simulink model "mw_spectrumanalyser"  (R2020a)
settings: Solver=VariableStepAuto  StartTime=0.0  StopTime=100000/256e6  RelTol=1e-3
InitFcn:
  | fs = 256e6;
undefined symbols (not defined in the file or in its folder): designMultirateFIR
libraries: hdlsllib x109, simulink x50, dsphdlxfrm x8, dspmlti4 x6, dspswit3 x4, dspsigops x2, dspsigattribs x2
(part 1 of 3)
settings Model: Creator=david  LastModifiedBy=david
settings OptimizationCC: BlockReduction=off  ConditionallyExecuteInputs=off  DefaultParameterBehavior=Inlined
settings DebuggingCC: AlgebraicLoopMsg=error
settings HardwareCC: ProdBitPerPointer=32  ProdBitPerSizeT=32  ProdBitPerPtrDiffT=32  ProdLargestAtomicFloat=None  ProdIntDivRoundTo=Undefined  ProdEndianess=Unspecified  ProdWordSize=32  ProdHWDeviceType=ASIC/FPGA->ASIC/FPGA  TargetBitPerPointer=64  TargetBitPerSizeT=64  TargetBitPerPtrDiffT=64  TargetLongLongMode=on  TargetIntDivRoundTo=Zero  TargetEndianess=LittleEndian  TargetWordSize=64  TargetHWDeviceType=Custom Processor->MATLAB Host Computer  ProdEqTarget=off

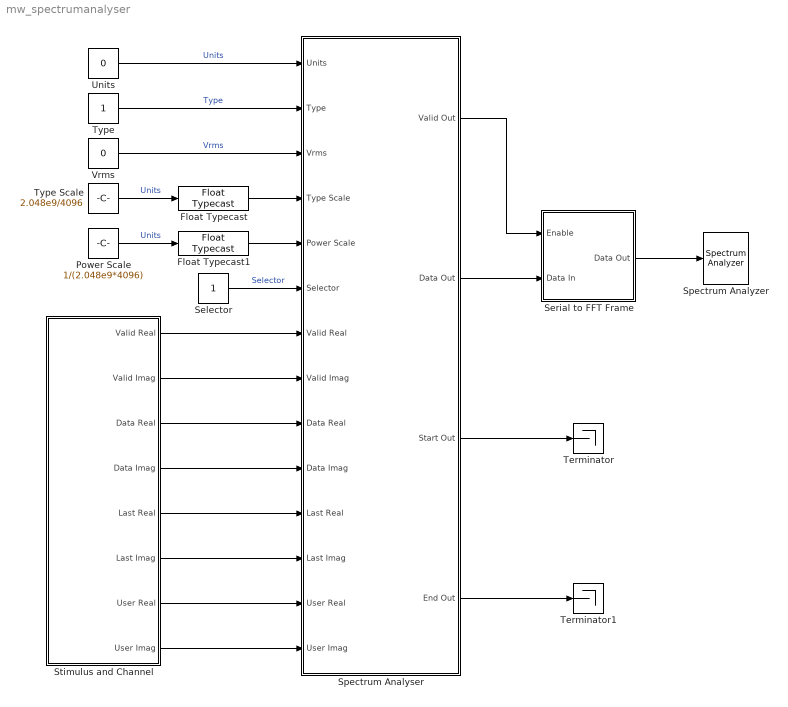
== system mw_spectrumanalyser ==
  Float Typecast : FloatTypecast
  Float Typecast1 : FloatTypecast
  Power Scale : Constant  Value=1/(2.048e9*4096)  OutDataTypeStr=single  SampleTime=-1
  Selector : Constant  OutDataTypeStr=uint32  SampleTime=-1
  Serial to FFT Frame : Subsystem  mask{N=4096}
      mask prompts: N "FFT Size:"
      mask DialogControl DescGroupVar Prompt: Serial to FFT Frame
      mask DialogControl DescTextVar Prompt: This block converts serial FFT data to a frame of FFT data. An FFT shift is applied to correct for out of order FFT data.
      mask DialogControl ParameterGroupVar Prompt: Main
  Spectrum Analyzer : SpectrumAnalyzer  IsFrequencyInputMode=1
  Spectrum Analyser : Subsystem  TreatAsAtomicUnit=on
  Stimulus and Channel : Subsystem
  Terminator : Terminator
  Terminator1 : Terminator
  Type : Constant  OutDataTypeStr=uint32  SampleTime=-1
  Type Scale : Constant  Value=2.048e9/4096  OutDataTypeStr=single  SampleTime=-1
  Units : Constant  Value=0  OutDataTypeStr=uint32  SampleTime=-1
  Vrms : Constant  Value=0  OutDataTypeStr=uint32  SampleTime=-1
  wires:
  Spectrum Analyser/3(Start Out) -> Terminator/1
  Spectrum Analyser/4(End Out) -> Terminator1/1
  Spectrum Analyser/2(Data Out) -> Serial to FFT Frame/2(Data In)
  Spectrum Analyser/1(Valid Out) -> Serial to FFT Frame/1(Enable)
  Serial to FFT Frame/1(Data Out) -> Spectrum Analyzer/1
  Stimulus and Channel/1(Valid Real) -> Spectrum Analyser/7(Valid Real)
  Stimulus and Channel/2(Valid Imag) -> Spectrum Analyser/8(Valid Imag)
  Stimulus and Channel/3(Data Real) -> Spectrum Analyser/9(Data Real)
  Stimulus and Channel/4(Data Imag) -> Spectrum Analyser/10(Data Imag)
  Vrms/1 -> Spectrum Analyser/3(Vrms)  "Vrms"
  Type/1 -> Spectrum Analyser/2(Type)  "Type"
  Units/1 -> Spectrum Analyser/1(Units)  "Units"
  Type Scale/1 -> Float Typecast/1  "Units"
  Float Typecast/1 -> Spectrum Analyser/4(Type Scale)
  Float Typecast1/1 -> Spectrum Analyser/5(Power Scale)
  Power Scale/1 -> Float Typecast1/1  "Units"
  Stimulus and Channel/5(Last Real) -> Spectrum Analyser/11(Last Real)
  Stimulus and Channel/6(Last Imag) -> Spectrum Analyser/12(Last Imag)
  Stimulus and Channel/7(User Real) -> Spectrum Analyser/13(User Real)
  Stimulus and Channel/8(User Imag) -> Spectrum Analyser/14(User Imag)
  Selector/1 -> Spectrum Analyser/6(Selector)  "Selector"

== system mw_spectrumanalyser/Serial to FFT Frame ==
  Enable : Inport
  Data In : Inport  Port=2
  Enabled Subsystem2 : Subsystem  TreatAsAtomicUnit=on
  Float Typecast : FloatTypecast
  Matrix Concatenate2 : Concatenate  Mode=Multidimensional array
  Selector1 : Selector  InputPortWidth=N  IndexOptions=Index vector (dialog)  Indices=[1:1:N/2+1]  OutputSizes=1
  Selector4 : Selector  InputPortWidth=N  IndexOptions=Index vector (dialog)  Indices=[N/2+2:1:N]  OutputSizes=1
  Data Out : Outport
  wires:
  Float Typecast/1 -> Data Out/1
  Selector4/1 -> Matrix Concatenate2/1
  Selector1/1 -> Matrix Concatenate2/2
  Matrix Concatenate2/1 -> Float Typecast/1
  Data In/1 -> Enabled Subsystem2/1(Data In)
  Enable/1 -> Enabled Subsystem2/Enable
  Enabled Subsystem2/1(Data Out) -> Selector1/1, Selector4/1

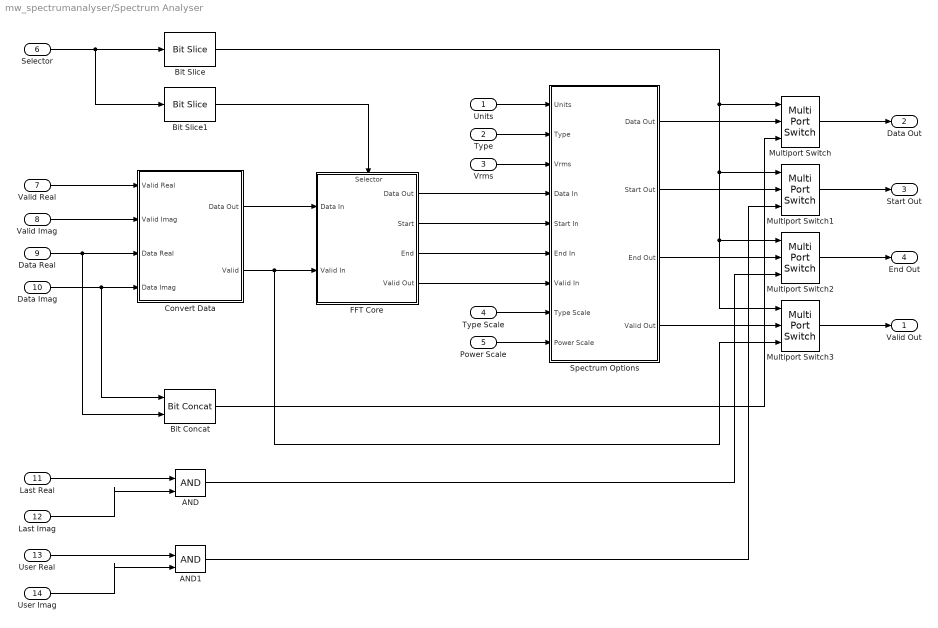
== system mw_spectrumanalyser/Spectrum Analyser ==
  Units : Inport
  Type : Inport  Port=2
  Vrms : Inport  Port=3
  Type Scale : Inport  Port=4
  Power Scale : Inport  Port=5
  Selector : Inport  Port=6
  Valid Real : Inport  Port=7
  Valid Imag : Inport  Port=8
  Data Real : Inport  Port=9
  Data Imag : Inport  Port=10
  Last Real : Inport  Port=11
  Last Imag : Inport  Port=12
  User Real : Inport  Port=13
  User Imag : Inport  Port=14
  AND : Logic  IconShape=distinctive  AllPortsSameDT=off  OutDataTypeStr=boolean
  AND1 : Logic  IconShape=distinctive  AllPortsSameDT=off  OutDataTypeStr=boolean
  Bit Concat : hdlsllib/Logic and Bit Operations/Bit Concat  numInputs=2
  Bit Slice : hdlsllib/Logic and Bit Operations/Bit Slice  lidx=8  ridx=8
      settings: SourceProductBaseCode=SL
  Bit Slice1 : hdlsllib/Logic and Bit Operations/Bit Slice  lidx=7  ridx=0
      settings: SourceProductBaseCode=SL
  Convert Data : Subsystem
  FFT Core : Subsystem  VariantControl=FFT
      settings: PortSchema="{\"entries\":[{\"content\":{\"sides\":[{\"content\":{\"connectorIds\":[\"In1\",\"In2\"]},\"type\":\"ConnectorPlacement.EquallySpacedRectSide\",\"uuid\":\"5a82c6db-67e2-4b0c-874b-00e78ac3fdee\"},{\"content\":{\"connectorIds\":[\"Out1\",\"Out2\",\"Out3\",\"Out4\"],\"side\":\"RIGHT\"},\"type\":\"ConnectorPlacement.EquallySpacedRectSide\",\"uuid\":\"dd11d034-f57b-4257-86c3-a224676007d8\"},{\"content\":{\"connectorIds\":[\"In3\"],\"side\":\"TOP\"},\"type\":\"ConnectorPlacement.EquallySpacedRectSide\",\"uuid\":\"15a5b623-5fad-4b26-a0b8-0856d140e740\"}]},\"type\":\"ConnectorPlacement.EquallySpacedConnector\",\"uuid\":\"f1901d0a-924b-44ce-aa2b-38fba4da21f9\"}],\"packageUris\":[\"http://schema.mathworks.com/mf0/Connector/19700101\"],\"version\":\"1.0\"}"
  Multiport Switch{,1..3} (4 alike) : MultiPortSwitch  DataPortOrder=Zero-based contiguous  Inputs=2  zeroidx=on
  Spectrum Options : Subsystem  VariantControl=Options
  Valid Out : Outport
  Data Out : Outport  Port=2
  Start Out : Outport  Port=3
  End Out : Outport  Port=4
  wires:
  FFT Core/4(Valid Out) -> Spectrum Options/7(Valid In)
  FFT Core/3(End) -> Spectrum Options/6(End In)
  FFT Core/2(Start) -> Spectrum Options/5(Start In)
  FFT Core/1(Data Out) -> Spectrum Options/4(Data In)
  Vrms/1 -> Spectrum Options/3(Vrms)
  Type/1 -> Spectrum Options/2(Type)
  Units/1 -> Spectrum Options/1(Units)
  Convert Data/1(Data Out) -> FFT Core/1(Data In)
  Data Imag/1 -> Bit Concat/1, Convert Data/4(Data Imag)
  Data Real/1 -> Bit Concat/2, Convert Data/3(Data Real)
  Valid Imag/1 -> Convert Data/2(Valid Imag)
  Valid Real/1 -> Convert Data/1(Valid Real)
  Type Scale/1 -> Spectrum Options/8(Type Scale)
  Power Scale/1 -> Spectrum Options/9(Power Scale)
  Spectrum Options/1(Data Out) -> Multiport Switch/2
  Multiport Switch/1 -> Data Out/1
  Spectrum Options/2(Start Out) -> Multiport Switch1/2
  Multiport Switch1/1 -> Start Out/1
  Spectrum Options/3(End Out) -> Multiport Switch2/2
  Multiport Switch2/1 -> End Out/1
  Spectrum Options/4(Valid Out) -> Multiport Switch3/2
  Multiport Switch3/1 -> Valid Out/1
  Selector/1 -> Bit Slice1/1, Bit Slice/1
  Last Real/1 -> AND/1
  Last Imag/1 -> AND/2
  User Real/1 -> AND1/1
  User Imag/1 -> AND1/2
  Bit Slice/1 -> Multiport Switch3/1, Multiport Switch2/1, Multiport Switch1/1, Multiport Switch/1
  Bit Concat/1 -> Multiport Switch/3
  Convert Data/2(Valid) -> Multiport Switch3/3, FFT Core/2(Valid In)
  AND/1 -> Multiport Switch2/3
  AND1/1 -> Multiport Switch1/3
  Bit Slice1/1 -> FFT Core/3(Selector)

== system mw_spectrumanalyser/Stimulus and Channel ==
  Channel : Subsystem
  Enable : Constant  OutDataTypeStr=boolean  SampleTime=-1
  Packet Size : Constant  Value=512  OutDataTypeStr=uint32  SampleTime=-1
  SSR Mode : Constant  Value=3  OutDataTypeStr=uint32  SampleTime=-1
  SSR Subset Converter Im : Subsystem  TreatAsAtomicUnit=on
  SSR Subset Converter Re : Subsystem  TreatAsAtomicUnit=on
  Transmitter : Subsystem  TreatAsAtomicUnit=on
  Value : Constant  Value=hex2dec('7FFF7FFF')  OutDataTypeStr=uint32  SampleTime=-1
  Valid Real : Outport
  Valid Imag : Outport  Port=2
  Data Real : Outport  Port=3
  Data Imag : Outport  Port=4
  Last Real : Outport  Port=5
  Last Imag : Outport  Port=6
  User Real : Outport  Port=7
  User Imag : Outport  Port=8
  wires:
  Enable/1 -> Transmitter/1(Enable)  "Enable"
  Transmitter/1(Valid) -> Channel/1(Valid)
  Transmitter/2(Data) -> Channel/2(Data)
  Value/1 -> Transmitter/2(Value)  "Value"
  Channel/2(Data Real) -> SSR Subset Converter Re/4(Data In)
  Channel/1(Valid Real) -> SSR Subset Converter Re/3(Valid In)
  SSR Mode/1 -> SSR Subset Converter Im/2(SSR Mode), SSR Subset Converter Re/2(SSR Mode)
  Packet Size/1 -> SSR Subset Converter Im/1(Packet Size), SSR Subset Converter Re/1(Packet Size)
  SSR Subset Converter Re/1(Valid Out) -> Valid Real/1
  SSR Subset Converter Re/2(Data Out) -> Data Real/1
  SSR Subset Converter Im/2(Data Out) -> Data Imag/1
  SSR Subset Converter Im/1(Valid Out) -> Valid Imag/1
  Channel/3(Valid Imag) -> SSR Subset Converter Im/3(Valid In)
  Channel/4(Data Imag) -> SSR Subset Converter Im/4(Data In)
  SSR Subset Converter Re/4(Last Out) -> Last Real/1
  SSR Subset Converter Im/4(Last Out) -> Last Imag/1
  SSR Subset Converter Re/3(User Out) -> User Real/1
  SSR Subset Converter Im/3(User Out) -> User Imag/1

== system mw_spectrumanalyser/Serial to FFT Frame/Enabled Subsystem2 ==
  Data In : Inport
  Enable : EnablePort
  Buffer : Buffer  N=N  OutputFrames=off
  Data Out : Outport
  wires:
  Buffer/1 -> Data Out/1
  Data In/1 -> Buffer/1

== system mw_spectrumanalyser/Spectrum Analyser/Convert Data ==
  Valid Real : Inport
  Valid Imag : Inport  Port=2
  Data Real : Inport  Port=3
  Data Imag : Inport  Port=4
  AND : Logic  IconShape=distinctive  AllPortsSameDT=off  OutDataTypeStr=boolean
  Data Type Conversion : DataTypeConversion  OutDataTypeStr=fixdt(1,16,15)  ConvertRealWorld=Stored Integer (SI)
  Data Type Conversion1 : DataTypeConversion  OutDataTypeStr=fixdt(1,16,15)  ConvertRealWorld=Stored Integer (SI)
  Real-Imag to Complex : RealImagToComplex
  Data Out : Outport
  Valid : Outport  Port=2
  wires:
  Real-Imag to Complex/1 -> Data Out/1
  AND/1 -> Valid/1
  Valid Real/1 -> AND/1
  Data Imag/1 -> Data Type Conversion1/1
  Data Type Conversion/1 -> Real-Imag to Complex/1
  Data Real/1 -> Data Type Conversion/1
  Data Type Conversion1/1 -> Real-Imag to Complex/2
  Valid Imag/1 -> AND/2

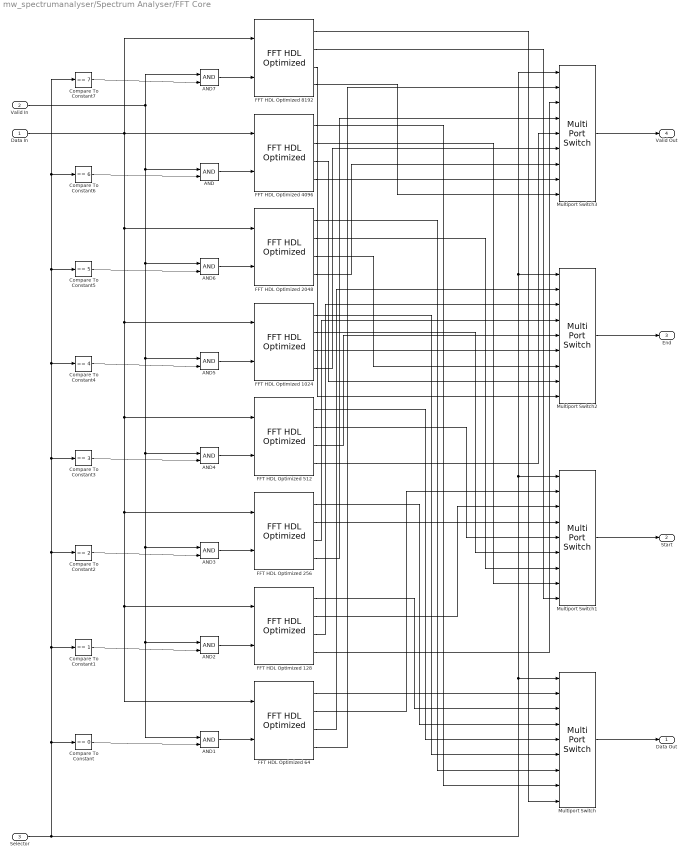
== system mw_spectrumanalyser/Spectrum Analyser/FFT Core ==
  Data In : Inport
  Valid In : Inport  Port=2
  Selector : Inport  Port=3
  AND{,1..7} (8 alike) : Logic  IconShape=distinctive  AllPortsSameDT=off  OutDataTypeStr=boolean
  Compare To Constant : simulink/Logic and Bit Operations/Compare To Constant  relop===  const=0  OutDataTypeStr=boolean
  Compare To Constant1 : simulink/Logic and Bit Operations/Compare To Constant  relop===  const=1  OutDataTypeStr=boolean
  Compare To Constant2 : simulink/Logic and Bit Operations/Compare To Constant  relop===  const=2  OutDataTypeStr=boolean
  Compare To Constant3 : simulink/Logic and Bit Operations/Compare To Constant  relop===  const=3  OutDataTypeStr=boolean
  Compare To Constant4 : simulink/Logic and Bit Operations/Compare To Constant  relop===  const=4  OutDataTypeStr=boolean
  Compare To Constant5 : simulink/Logic and Bit Operations/Compare To Constant  relop===  const=5  OutDataTypeStr=boolean
  Compare To Constant6 : simulink/Logic and Bit Operations/Compare To Constant  relop===  const=6  OutDataTypeStr=boolean
  Compare To Constant7 : simulink/Logic and Bit Operations/Compare To Constant  relop===  const=7  OutDataTypeStr=boolean
  FFT HDL Optimized 1024 : dsphdlxfrm/FFT HDL Optimized  FFTLength=1024  Architecture=Streaming Radix 2^2  ComplexMultiplication=Use 4 multipliers and 2 adders  BitReversedOutput=off  BitReversedInput=off  Normalize=off  SimulateUsing=Code generation  RoundingMethod=Round  ResetInputPort=off  StartOutputPort=on  EndOutputPort=on
      settings: SourceProductBaseCode=DS
  FFT HDL Optimized 128 : dsphdlxfrm/FFT HDL Optimized  FFTLength=128  Architecture=Streaming Radix 2^2  ComplexMultiplication=Use 4 multipliers and 2 adders  BitReversedOutput=off  BitReversedInput=off  Normalize=off  SimulateUsing=Code generation  RoundingMethod=Round  ResetInputPort=off  StartOutputPort=on  EndOutputPort=on
      settings: SourceProductBaseCode=DS
  FFT HDL Optimized 2048 : dsphdlxfrm/FFT HDL Optimized  FFTLength=2048  Architecture=Streaming Radix 2^2  ComplexMultiplication=Use 4 multipliers and 2 adders  BitReversedOutput=off  BitReversedInput=off  Normalize=off  SimulateUsing=Code generation  RoundingMethod=Round  ResetInputPort=off  StartOutputPort=on  EndOutputPort=on
      settings: SourceProductBaseCode=DS
  FFT HDL Optimized 256 : dsphdlxfrm/FFT HDL Optimized  FFTLength=256  Architecture=Streaming Radix 2^2  ComplexMultiplication=Use 4 multipliers and 2 adders  BitReversedOutput=off  BitReversedInput=off  Normalize=off  SimulateUsing=Code generation  RoundingMethod=Round  ResetInputPort=off  StartOutputPort=on  EndOutputPort=on
      settings: SourceProductBaseCode=DS
  FFT HDL Optimized 4096 : dsphdlxfrm/FFT HDL Optimized  FFTLength=4096  Architecture=Streaming Radix 2^2  ComplexMultiplication=Use 4 multipliers and 2 adders  BitReversedOutput=off  BitReversedInput=off  Normalize=off  SimulateUsing=Code generation  RoundingMethod=Round  ResetInputPort=off  StartOutputPort=on  EndOutputPort=on
      settings: SourceProductBaseCode=DS
  FFT HDL Optimized 512 : dsphdlxfrm/FFT HDL Optimized  FFTLength=512  Architecture=Streaming Radix 2^2  ComplexMultiplication=Use 4 multipliers and 2 adders  BitReversedOutput=off  BitReversedInput=off  Normalize=off  SimulateUsing=Code generation  RoundingMethod=Round  ResetInputPort=off  StartOutputPort=on  EndOutputPort=on
      settings: SourceProductBaseCode=DS
  FFT HDL Optimized 64 : dsphdlxfrm/FFT HDL Optimized  FFTLength=64  Architecture=Streaming Radix 2^2  ComplexMultiplication=Use 4 multipliers and 2 adders  BitReversedOutput=off  BitReversedInput=off  Normalize=off  SimulateUsing=Code generation  RoundingMethod=Round  ResetInputPort=off  StartOutputPort=on  EndOutputPort=on
      settings: SourceProductBaseCode=DS
  FFT HDL Optimized 8192 : dsphdlxfrm/FFT HDL Optimized  FFTLength=8192  Architecture=Streaming Radix 2^2  ComplexMultiplication=Use 4 multipliers and 2 adders  BitReversedOutput=off  BitReversedInput=off  Normalize=off  SimulateUsing=Code generation  RoundingMethod=Round  ResetInputPort=off  StartOutputPort=on  EndOutputPort=on
      settings: SourceProductBaseCode=DS
  Multiport Switch{,1..3} (4 alike) : MultiPortSwitch  DataPortOrder=Zero-based contiguous  Inputs=8  zeroidx=on
  Data Out : Outport
  Start : Outport  Port=2
  End : Outport  Port=3
  Valid Out : Outport  Port=4
  wires:
  AND/1 -> FFT HDL Optimized 4096/2
  AND1/1 -> FFT HDL Optimized 64/2
  Compare To Constant/1 -> AND1/2
  Selector/1 -> Multiport Switch3/1, Multiport Switch2/1, Multiport Switch1/1, Multiport Switch/1, Compare To Constant7/1, Compare To Constant6/1, Compare To Constant5/1, Compare To Constant4/1, Compare To Constant3/1, Compare To Constant2/1, Compare To Constant1/1, Compare To Constant/1
  Valid In/1 -> AND7/1, AND/1, AND6/1, AND5/1, AND4/1, AND3/1, AND2/1, AND1/1
  AND3/1 -> FFT HDL Optimized 256/2
  AND2/1 -> FFT HDL Optimized 128/2
  AND4/1 -> FFT HDL Optimized 512/2
  AND5/1 -> FFT HDL Optimized 1024/2
  AND6/1 -> FFT HDL Optimized 2048/2
  AND7/1 -> FFT HDL Optimized 8192/2
  Compare To Constant7/1 -> AND7/2
  Data In/1 -> FFT HDL Optimized 64/1, FFT HDL Optimized 128/1, FFT HDL Optimized 256/1, FFT HDL Optimized 512/1, FFT HDL Optimized 1024/1, FFT HDL Optimized 2048/1, FFT HDL Optimized 4096/1, FFT HDL Optimized 8192/1
  Compare To Constant1/1 -> AND2/2
  Compare To Constant2/1 -> AND3/2
  Compare To Constant3/1 -> AND4/2
  Compare To Constant4/1 -> AND5/2
  Compare To Constant5/1 -> AND6/2
  Compare To Constant6/1 -> AND/2
  FFT HDL Optimized 64/1 -> Multiport Switch/2
  FFT HDL Optimized 128/1 -> Multiport Switch/3
  FFT HDL Optimized 256/1 -> Multiport Switch/4
  FFT HDL Optimized 512/1 -> Multiport Switch/5
  FFT HDL Optimized 1024/1 -> Multiport Switch/6
  FFT HDL Optimized 2048/1 -> Multiport Switch/7
  FFT HDL Optimized 4096/1 -> Multiport Switch/8
  FFT HDL Optimized 8192/1 -> Multiport Switch/9
  FFT HDL Optimized 256/2 -> Multiport Switch1/4
  FFT HDL Optimized 64/2 -> Multiport Switch1/2
  FFT HDL Optimized 128/2 -> Multiport Switch1/3
  FFT HDL Optimized 512/2 -> Multiport Switch1/5
  FFT HDL Optimized 1024/2 -> Multiport Switch1/6
  FFT HDL Optimized 2048/2 -> Multiport Switch1/7
  FFT HDL Optimized 4096/2 -> Multiport Switch1/8
  FFT HDL Optimized 8192/2 -> Multiport Switch1/9
  FFT HDL Optimized 1024/3 -> Multiport Switch2/6
  FFT HDL Optimized 512/3 -> Multiport Switch2/5
  FFT HDL Optimized 256/3 -> Multiport Switch2/4
  FFT HDL Optimized 2048/3 -> Multiport Switch2/7
  FFT HDL Optimized 4096/3 -> Multiport Switch2/8
  FFT HDL Optimized 8192/3 -> Multiport Switch2/9
  FFT HDL Optimized 128/3 -> Multiport Switch2/3
  FFT HDL Optimized 64/3 -> Multiport Switch2/2
  FFT HDL Optimized 4096/4 -> Multiport Switch3/8
  FFT HDL Optimized 8192/4 -> Multiport Switch3/9
  FFT HDL Optimized 2048/4 -> Multiport Switch3/7
  FFT HDL Optimized 1024/4 -> Multiport Switch3/6
  FFT HDL Optimized 512/4 -> Multiport Switch3/5
  FFT HDL Optimized 256/4 -> Multiport Switch3/4
  FFT HDL Optimized 128/4 -> Multiport Switch3/3
  FFT HDL Optimized 64/4 -> Multiport Switch3/2
  Multiport Switch3/1 -> Valid Out/1
  Multiport Switch2/1 -> End/1
  Multiport Switch1/1 -> Start/1
  Multiport Switch/1 -> Data Out/1

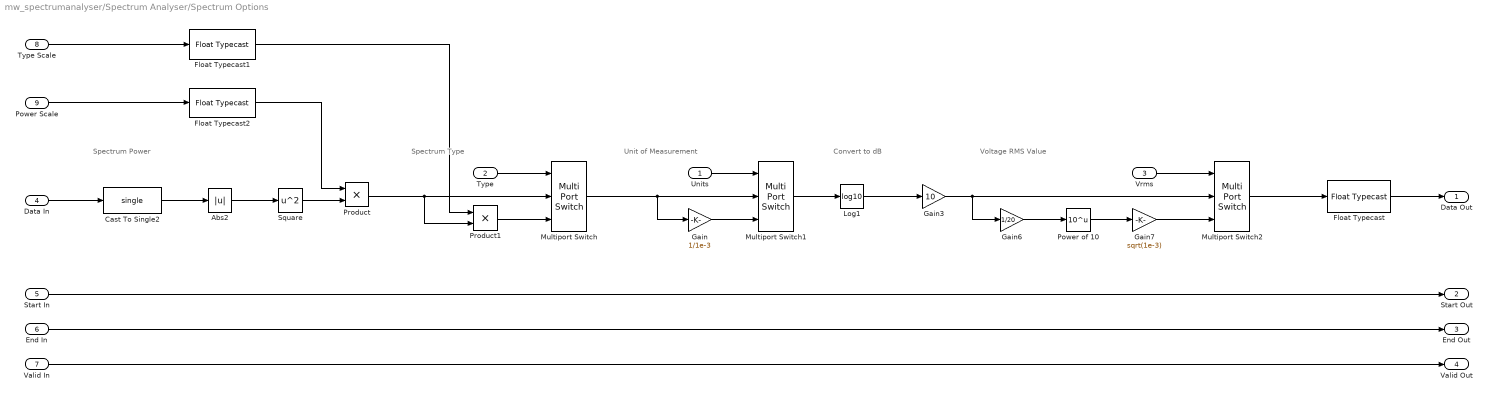
== system mw_spectrumanalyser/Spectrum Analyser/Spectrum Options ==
  note: Spectrum Power
  note: Spectrum Type
  note: Unit of Measurement
  note: Convert to dB
  note: Voltage RMS Value
  Units : Inport
  Type : Inport  Port=2
  Vrms : Inport  Port=3
  Data In : Inport  Port=4
  Start In : Inport  Port=5
  End In : Inport  Port=6
  Valid In : Inport  Port=7
  Type Scale : Inport  Port=8
  Power Scale : Inport  Port=9
  Abs2 : Abs
  Cast To Single2 : DataTypeConversion  OutDataTypeStr=single
  Float Typecast : FloatTypecast
  Float Typecast1 : FloatTypecast
  Float Typecast2 : FloatTypecast
  Gain : Gain  Gain=1/1e-3
  Gain3 : Gain  Gain=10  ParamDataTypeStr=single  OutDataTypeStr=single
  Gain6 : Gain  Gain=1/20
  Gain7 : Gain  Gain=sqrt(1e-3)
  Log1 : Math  Operator=log10  SignedPower=on  SaturateOnIntegerOverflow=on
  Multiport Switch : MultiPortSwitch  DataPortOrder=Zero-based contiguous  Inputs=2  zeroidx=on
  Multiport Switch1 : MultiPortSwitch  DataPortOrder=Zero-based contiguous  Inputs=2  zeroidx=on
  Multiport Switch2 : MultiPortSwitch  DataPortOrder=Zero-based contiguous  Inputs=2  zeroidx=on
  Power of 10 : Math  Operator=10^u  SaturateOnIntegerOverflow=on
  Product : Product
  Product1 : Product
  Square : Math  Operator=square  SaturateOnIntegerOverflow=on
  Data Out : Outport
  Start Out : Outport  Port=2
  End Out : Outport  Port=3
  Valid Out : Outport  Port=4
  wires:
  Valid In/1 -> Valid Out/1
  End In/1 -> End Out/1
  Float Typecast/1 -> Data Out/1
  Vrms/1 -> Multiport Switch2/1
  Units/1 -> Multiport Switch1/1
  Type/1 -> Multiport Switch/1
  Product1/1 -> Multiport Switch/3
  Gain/1 -> Multiport Switch1/3
  Gain7/1 -> Multiport Switch2/3
  Multiport Switch2/1 -> Float Typecast/1
  Gain3/1 -> Gain6/1, Multiport Switch2/2
  Power of 10/1 -> Gain7/1
  Gain6/1 -> Power of 10/1
  Multiport Switch1/1 -> Log1/1
  Multiport Switch/1 -> Gain/1, Multiport Switch1/2
  Log1/1 -> Gain3/1
  Start In/1 -> Start Out/1
  Cast To Single2/1 -> Abs2/1
  Data In/1 -> Cast To Single2/1
  Product/1 -> Product1/2, Multiport Switch/2
  Abs2/1 -> Square/1
  Square/1 -> Product/2
  Type Scale/1 -> Float Typecast1/1
  Power Scale/1 -> Float Typecast2/1
  Float Typecast1/1 -> Product1/1
  Float Typecast2/1 -> Product/1

== system mw_spectrumanalyser/Stimulus and Channel/Channel ==
  Valid : Inport
  Data : Inport  Port=2
  RF-ADC : Subsystem  mask{fs_ghz=4.096, decim=2x, ssr=8, mode=Fine, fc=0.256, fph=0, fcoarse=fs/4}
      mask prompts: fs_ghz "Sample Rate (GHz):"; decim "Interpolation Mode:"; ssr "Samples per AXI4-Stream Cycle:"; mode "Mixer Type:"; fc "NCO Frequency (GHz):"; fph "NCO Phase (Rads):"; fcoarse "Frequency:"
      mask init:
      | % Obtain the sample rate in Hz
      | fs = str2double(get_param(gcb, 'fs_ghz'))*1e9;
      | 
      | % Set the mode of the RF-DAC interpolation filter
      | switch get_param(gcb, 'decim')
      |     case '1x'
      |         D = 1;
      |     case '2x'
      |         D = 2;
      |     case '4x'
      |         D = 4;
      |     case '8x'
      |         D = 8;
      |     otherwise
      |         D = 1;
      | end
      | 
      | % Get the AXI-Stream clock for display to user
      | axi_clk = (fs/(str2double(get_param(gcb, 'ssr'))*D))*1e-6;
      | 
      | % Get the block mask object to manipulate settings
      | mo = get_param(gcb, 'MaskObject');
      | 
      | % Update text to display the required AXI-Stream clock
      | tc = mo.getDialogControl('axi_text');
      | tc.Prompt = ['      Required AXI-Stream Clock: ', num2str(axi_clk), ' MHz'];
      | 
      | % Set the RF-DAC Mixer mode
      | switch get_param(gcb, 'mode')
      |     case 'Bypass'
      |         m = 0;
      |     case 'Coarse'
      |         m = 1;
      |     case 'Fine'
      |         m = 2;
      |     otherwise
      |         m = 0;
      | end
      | 
      | % Set the RF-DAC Coarse Mixer mode
      | switch get_param(gcb, 'fcoarse')
      |     case 'fs/2'
      |         mc = 0;
      |     case 'fs/4'
      |         mc = 1;
      |     case '-fs/4'
      |         mc = 2;
      |     otherwise
      |         mc = 0;
      | end
      | 
      | % Set other blocks
      | set_param([gcb, '/Decimation Filter'], 'decim', get_param(gcb, 'decim'));
      mask Callback fs_ghz:
      | % Obtain the sample rate in Hz
      | fs = str2double(get_param(gcb, 'fs_ghz'))*1e9;
      | 
      | % Set the mode of the RF-DAC interpolation filter
      | switch get_param(gcb, 'decim')
      |     case '1x'
      |         D = 1;
      |     case '2x'
      |         D = 2;
      |     case '4x'
      |         D = 4;
      |     case '8x'
      |         D = 8;
      |     otherwise
      |         D = 1;
      | end
      | 
      | % Get the AXI-Stream clock for display to user
      | axi_clk = (fs/(str2double(get_param(gcb, 'ssr'))*D))*1e-6;
      | 
      | % Get the block mask object to manipulate settings
      | mo = get_param(gcb, 'MaskObject');
      | 
      | % Update text to display the required AXI-Stream clock
      | tc = mo.getDialogControl('axi_text');
      | tc.Prompt = ['      Required AXI-Stream Clock: ', num2str(axi_clk), ' MHz'];
      mask TypeOptions decim: 1x | 2x | 4x | 8x
      mask Callback decim:
      | % Obtain the sample rate in Hz
      | fs = str2double(get_param(gcb, 'fs_ghz'))*1e9;
      | 
      | % Set the mode of the RF-DAC interpolation filter
      | switch get_param(gcb, 'decim')
      |     case '1x'
      |         D = 1;
      |     case '2x'
      |         D = 2;
      |     case '4x'
      |         D = 4;
      |     case '8x'
      |         D = 8;
      |     otherwise
      |         D = 1;
      | end
      | 
      | % Get the AXI-Stream clock for display to user
      | axi_clk = (fs/(str2double(get_param(gcb, 'ssr'))*D))*1e-6;
      | 
      | % Get the block mask object to manipulate settings
      | mo = get_param(gcb, 'MaskObject');
      | 
      | % Update text to display the required AXI-Stream clock
      | tc = mo.getDialogControl('axi_text');
      | tc.Prompt = ['      Required AXI-Stream Clock: ', num2str(axi_clk), ' MHz'];
      mask TypeOptions ssr: 1 | 2 | 3 | 4 | 5 | 6 | 7 | 8 | 9 | 10 | 11 | 12 | 13 | 14 | 15 | 16
      mask Callback ssr:
      | % Obtain the sample rate in Hz
      | fs = str2double(get_param(gcb, 'fs_ghz'))*1e9;
      | 
      | % Set the mode of the RF-DAC interpolation filter
      | switch get_param(gcb, 'decim')
      |     case '1x'
      |         D = 1;
      |     case '2x'
      |         D = 2;
      |     case '4x'
      |         D = 4;
      |     case '8x'
      |         D = 8;
      |     otherwise
      |         D = 1;
      | end
      | 
      | % Get the AXI-Stream clock for display to user
      | axi_clk = (fs/(str2double(get_param(gcb, 'ssr'))*D))*1e-6;
      | 
      | % Get the block mask object to manipulate settings
      | mo = get_param(gcb, 'MaskObject');
      | 
      | % Update text to display the required AXI-Stream clock
      | tc = mo.getDialogControl('axi_text');
      | tc.Prompt = ['      Required AXI-Stream Clock: ', num2str(axi_clk), ' MHz'];
      mask TypeOptions mode: Coarse | Fine
      mask Callback mode:
      | % Get the block mask object to manipulate settings
      | mo = get_param(gcb, 'MaskObject');
      | 
      | % Hide group depending on Mixer mode choice
      | switch get_param(gcb, 'mode')
      |     case 'Bypass'
      |         mo.getDialogControl('coarse_group').Visible='off';
      |         mo.getDialogControl('mixer_group').Visible='off';
      |     case 'Coarse'
      |         mo.getDialogControl('coarse_group').Visible='on';
      |         mo.getDialogControl('mixer_group').Visible='off';
      |     case 'Fine'
      |         mo.getDialogControl('coarse_group').Visible='off';
      |         mo.getDialogControl('mixer_group').Visible='on';
      |     otherwise
      |         mo.getDialogControl('coarse_group').Visible='off';
      |         mo.getDialogControl('mixer_group').Visible='off';
      | end
      mask TypeOptions fcoarse: fs/2 | fs/4 | -fs/4
      mask DialogControl DescGroupVar Prompt: RF-DAC
      mask DialogControl DescTextVar Prompt: This block simulates one RF-ADC channel.
      mask DialogControl main_group Prompt: Data Settings
      mask DialogControl axi_text Prompt: Required AXI-Stream Clock: 256 MHz
      mask DialogControl Container5 Prompt: Mixer Settings
  RF-DAC : Subsystem  mask{fs_ghz=4.096, interp=4x, ssr=4, mode=Fine, fc=0.512, fph=0, fcoarse=fs/4}
      mask prompts: fs_ghz "Sample Rate (GHz):"; interp "Interpolation Mode:"; ssr "Samples per AXI4-Stream Cycle:"; mode "Mixer Type:"; fc "NCO Frequency (GHz):"; fph "NCO Phase (Rads):"; fcoarse "Frequency:"
      mask init:
      | % Obtain the sample rate in Hz
      | fs = str2double(get_param(gcb, 'fs_ghz'))*1e9;
      | 
      | % Set the mode of the RF-DAC interpolation filter
      | switch get_param(gcb, 'interp')
      |     case '1x'
      |         L = 1;
      |     case '2x'
      |         L = 2;
      |     case '4x'
      |         L = 4;
      |     case '8x'
      |         L = 8;
      |     otherwise
      |         L = 1;
      | end
      | 
      | % Get the AXI-Stream clock for display to user
      | axi_clk = (fs/(str2double(get_param(gcb, 'ssr'))*L))*1e-6;
      | 
      | % Get the block mask object to manipulate settings
      | mo = get_param(gcb, 'MaskObject');
      | 
      | % Update text to display the required AXI-Stream clock
      | tc = mo.getDialogControl('axi_text');
      | tc.Prompt = ['      Required AXI-Stream Clock: ', num2str(axi_clk), ' MHz'];
      | 
      | % Set the RF-DAC Mixer mode
      | switch get_param(gcb, 'mode')
      |     case 'Bypass'
      |         m = 0;
      |     case 'Coarse'
      |         m = 1;
      |     case 'Fine'
      |         m = 2;
      |     otherwise
      |         m = 0;
      | end
      | 
      | % Set the RF-DAC Coarse Mixer mode
      | switch get_param(gcb, 'fcoarse')
      |     case 'fs/2'
      |         mc = 0;
      |     case 'fs/4'
      |         mc = 1;
      |     case '-fs/4'
      |         mc = 2;
      |     otherwise
      |         mc = 0;
      | end
      | 
      | % Set other blocks
      | set_param([gcb, '/Interpolation Filter'], 'interp', get_param(gcb, 'interp'));
      mask Callback fs_ghz:
      | % Obtain the sample rate in Hz
      | fs = str2double(get_param(gcb, 'fs_ghz'))*1e9;
      | 
      | % Set the mode of the RF-DAC interpolation filter
      | switch get_param(gcb, 'interp')
      |     case '1x'
      |         L = 1;
      |     case '2x'
      |         L = 2;
      |     case '4x'
      |         L = 4;
      |     case '8x'
      |         L = 8;
      |     otherwise
      |         L = 1;
      | end
      | 
      | % Get the AXI-Stream clock for display to user
      | axi_clk = (fs/(str2double(get_param(gcb, 'ssr'))*L))*1e-6;
      | 
      | % Get the block mask object to manipulate settings
      | mo = get_param(gcb, 'MaskObject');
      | 
      | % Update text to display the required AXI-Stream clock
      | tc = mo.getDialogControl('axi_text');
      | tc.Prompt = ['      Required AXI-Stream Clock: ', num2str(axi_clk), ' MHz'];
      mask TypeOptions interp: 1x | 2x | 4x | 8x
      mask Callback interp:
      | % Obtain the sample rate in Hz
      | fs = str2double(get_param(gcb, 'fs_ghz'))*1e9;
      | 
      | % Set the mode of the RF-DAC interpolation filter
      | switch get_param(gcb, 'interp')
      |     case '1x'
      |         L = 1;
      |     case '2x'
      |         L = 2;
      |     case '4x'
      |         L = 4;
      |     case '8x'
      |         L = 8;
      |     otherwise
      |         L = 1;
      | end
      | 
      | % Get the AXI-Stream clock for display to user
      | axi_clk = (fs/(str2double(get_param(gcb, 'ssr'))*L))*1e-6;
      | 
      | % Get the block mask object to manipulate settings
      | mo = get_param(gcb, 'MaskObject');
      | 
      | % Update text to display the required AXI-Stream clock
      | tc = mo.getDialogControl('axi_text');
      | tc.Prompt = ['      Required AXI-Stream Clock: ', num2str(axi_clk), ' MHz'];
      mask TypeOptions ssr: 1 | 2 | 3 | 4 | 5 | 6 | 7 | 8 | 9 | 10 | 11 | 12 | 13 | 14 | 15 | 16
      mask Callback ssr:
      | % Obtain the sample rate in Hz
      | fs = str2double(get_param(gcb, 'fs_ghz'))*1e9;
      | 
      | % Set the mode of the RF-DAC interpolation filter
      | switch get_param(gcb, 'interp')
      |     case '1x'
      |         L = 1;
      |     case '2x'
      |         L = 2;
      |     case '4x'
      |         L = 4;
      |     case '8x'
      |         L = 8;
      |     otherwise
      |         L = 1;
      | end
      | 
      | % Get the AXI-Stream clock for display to user
      | axi_clk = (fs/(str2double(get_param(gcb, 'ssr'))*L))*1e-6;
      | 
      | % Get the block mask object to manipulate settings
      | mo = get_param(gcb, 'MaskObject');
      | 
      | % Update text to display the required AXI-Stream clock
      | tc = mo.getDialogControl('axi_text');
      | tc.Prompt = ['      Required AXI-Stream Clock: ', num2str(axi_clk), ' MHz'];
      mask TypeOptions mode: Coarse | Fine
      mask Callback mode:
      | % Get the block mask object to manipulate settings
      | mo = get_param(gcb, 'MaskObject');
      | 
      | % Hide group depending on Mixer mode choice
      | switch get_param(gcb, 'mode')
      |     case 'Bypass'
      |         mo.getDialogControl('coarse_group').Visible='off';
      |         mo.getDialogControl('mixer_group').Visible='off';
      |     case 'Coarse'
      |         mo.getDialogControl('coarse_group').Visible='on';
      |         mo.getDialogControl('mixer_group').Visible='off';
      |     case 'Fine'
      |         mo.getDialogControl('coarse_group').Visible='off';
      |         mo.getDialogControl('mixer_group').Visible='on';
      |     otherwise
      |         mo.getDialogControl('coarse_group').Visible='off';
      |         mo.getDialogControl('mixer_group').Visible='off';
      | end
      mask TypeOptions fcoarse: fs/2 | fs/4 | -fs/4
      mask DialogControl DescGroupVar Prompt: RF-DAC
      mask DialogControl DescTextVar Prompt: This block simulates one RF-DAC channel.
      mask DialogControl main_group Prompt: Data Settings
      mask DialogControl axi_text Prompt: Required AXI-Stream Clock: 256 MHz
      mask DialogControl Container5 Prompt: Mixer Settings
  RX RF Balun : Gain  Gain=1/2
  TX RF Balun : Gain  Gain=1/2
  Valid Real : Outport
  Data Real : Outport  Port=2
  Valid Imag : Outport  Port=3
  Data Imag : Outport  Port=4
  wires:
  TX RF Balun/1 -> RX RF Balun/1
  Valid/1 -> RF-DAC/1(Valid)
  RF-ADC/3(Data Real) -> Data Real/1
  RX RF Balun/1 -> RF-ADC/1(Data In)
  Data/1 -> RF-DAC/2(Data)
  RF-ADC/4(Data Imag) -> Data Imag/1
  RF-ADC/1(Valid Real) -> Valid Real/1
  RF-DAC/1(Data Out) -> TX RF Balun/1
  RF-ADC/2(Valid Imag) -> Valid Imag/1

== system mw_spectrumanalyser/Stimulus and Channel/SSR Subset Converter Im ==
  Packet Size : Inport
  SSR Mode : Inport  Port=2
  Valid In : Inport  Port=3
  Data In : Inport  Port=4
  Bit Slice : hdlsllib/Logic and Bit Operations/Bit Slice  lidx=3  ridx=0
      settings: SourceProductBaseCode=SL
  SSR Deserializer : Subsystem
  SSR Packet Generator : Subsystem
      settings: PortSchema="{\"entries\":[{\"content\":{\"sides\":[{\"content\":{\"connectorIds\":[\"In1\",\"In2\",\"In3\"]},\"type\":\"ConnectorPlacement.EquallySpacedRectSide\",\"uuid\":\"a59bbe9b-b017-421a-b59e-ccf8f0be8c6c\"},{\"content\":{\"connectorIds\":[\"Out1\",\"Out2\",\"Out3\",\"Out4\"],\"side\":\"RIGHT\"},\"type\":\"ConnectorPlacement.EquallySpacedRectSide\",\"uuid\":\"db28a192-666b-40ba-a3e6-dc552d532719\"},{\"content\":{\"connectorIds\":[\"In4\"],\"side\":\"TOP\"},\"type\":\"ConnectorPlacement.EquallySpacedRectSide\",\"uuid\":\"3e188adb-8196-4c2d-ad94-9c10f40ece47\"}]},\"type\":\"ConnectorPlacement.EquallySpacedConnector\",\"uuid\":\"a5800336-434d-4feb-8784-3c17a141dc8c\"}],\"packageUris\":[\"http://schema.mathworks.com/mf0/Connector/19700101\"],\"version\":\"1.0\"}"
  SSR Serializer : Subsystem
  Valid Out : Outport
  Data Out : Outport  Port=2
  User Out : Outport  Port=3
  Last Out : Outport  Port=4
  wires:
  Data In/1 -> SSR Serializer/3(Data In)
  SSR Serializer/2(Data Out) -> SSR Packet Generator/3(Data In)
  SSR Packet Generator/4(EoF Out) -> SSR Deserializer/4(EoF In)
  SSR Serializer/1(Valid Out) -> SSR Packet Generator/2(Valid In)
  SSR Deserializer/3(SoF Out) -> User Out/1
  Bit Slice/1 -> SSR Serializer/1(SSR Control), SSR Packet Generator/1(Frame Drop)
  SSR Packet Generator/1(Valid Out) -> SSR Deserializer/1(Valid In)
  Valid In/1 -> SSR Serializer/2(Valid In)
  SSR Packet Generator/3(SoF Out) -> SSR Deserializer/3(SoF In)
  SSR Packet Generator/2(Data Out) -> SSR Deserializer/2(Data In)
  SSR Deserializer/2(Data Out) -> Data Out/1
  SSR Mode/1 -> Bit Slice/1
  SSR Deserializer/1(Valid Out) -> Valid Out/1
  SSR Deserializer/4(EoL Out) -> Last Out/1
  Packet Size/1 -> SSR Packet Generator/4(Packet Size)

== system mw_spectrumanalyser/Stimulus and Channel/SSR Subset Converter Re ==
  Packet Size : Inport
  SSR Mode : Inport  Port=2
  Valid In : Inport  Port=3
  Data In : Inport  Port=4
  Bit Slice : hdlsllib/Logic and Bit Operations/Bit Slice  lidx=3  ridx=0
      settings: SourceProductBaseCode=SL
  SSR Deserializer : Subsystem
  SSR Packet Generator : Subsystem
      settings: PortSchema="{\"entries\":[{\"content\":{\"sides\":[{\"content\":{\"connectorIds\":[\"In1\",\"In2\",\"In3\"]},\"type\":\"ConnectorPlacement.EquallySpacedRectSide\",\"uuid\":\"a59bbe9b-b017-421a-b59e-ccf8f0be8c6c\"},{\"content\":{\"connectorIds\":[\"Out1\",\"Out2\",\"Out3\",\"Out4\"],\"side\":\"RIGHT\"},\"type\":\"ConnectorPlacement.EquallySpacedRectSide\",\"uuid\":\"db28a192-666b-40ba-a3e6-dc552d532719\"},{\"content\":{\"connectorIds\":[\"In4\"],\"side\":\"TOP\"},\"type\":\"ConnectorPlacement.EquallySpacedRectSide\",\"uuid\":\"3e188adb-8196-4c2d-ad94-9c10f40ece47\"}]},\"type\":\"ConnectorPlacement.EquallySpacedConnector\",\"uuid\":\"a5800336-434d-4feb-8784-3c17a141dc8c\"}],\"packageUris\":[\"http://schema.mathworks.com/mf0/Connector/19700101\"],\"version\":\"1.0\"}"
  SSR Serializer : Subsystem
  Valid Out : Outport
  Data Out : Outport  Port=2
  User Out : Outport  Port=3
  Last Out : Outport  Port=4
  wires:
  Packet Size/1 -> SSR Packet Generator/4(Packet Size)
  SSR Deserializer/4(EoL Out) -> Last Out/1
  SSR Deserializer/1(Valid Out) -> Valid Out/1
  SSR Mode/1 -> Bit Slice/1
  SSR Deserializer/2(Data Out) -> Data Out/1
  SSR Packet Generator/2(Data Out) -> SSR Deserializer/2(Data In)
  SSR Packet Generator/3(SoF Out) -> SSR Deserializer/3(SoF In)
  Valid In/1 -> SSR Serializer/2(Valid In)
  SSR Packet Generator/1(Valid Out) -> SSR Deserializer/1(Valid In)
  Bit Slice/1 -> SSR Packet Generator/1(Frame Drop), SSR Serializer/1(SSR Control)
  SSR Deserializer/3(SoF Out) -> User Out/1
  SSR Serializer/1(Valid Out) -> SSR Packet Generator/2(Valid In)
  SSR Packet Generator/4(EoF Out) -> SSR Deserializer/4(EoF In)
  SSR Serializer/2(Data Out) -> SSR Packet Generator/3(Data In)
  Data In/1 -> SSR Serializer/3(Data In)

== system mw_spectrumanalyser/Stimulus and Channel/Transmitter ==
  Enable : Inport
  Value : Inport  Port=2
  Transmitter : Subsystem  TreatAsAtomicUnit=on
  Valid : Outport
  Data : Outport  Port=2
  wires:
  Transmitter/2(Data) -> Data/1
  Transmitter/1(Valid) -> Valid/1
  Enable/1 -> Transmitter/1(Enable)
  Value/1 -> Transmitter/2(Value)

== system mw_spectrumanalyser/Stimulus and Channel/Channel/RF-ADC ==
  Data In : Inport
  Complex to Real-Imag : ComplexToRealImag
  Decimation Filter : Subsystem  mask{decim=2x}
      mask prompts: decim "Decimation Factor:"
      mask init:
      | fir0 = dsp.FIRDecimator('DecimationFactor', 2,...
      |                            'CoefficientsDataType', 'Custom',...
      |                            'CustomCoefficientsDataType', numerictype([], 16, 14),...
      |                            'FullPrecisionOverride', false,...
      |                            'OutputDataType', 'Custom',...
      |                            'CustomOutputDataType', numerictype([], 16, 15),...
      |                            'Numerator', [-6, 0 54, 0, -254, 0, 1230, 2048, 1230, 0, -254, 0, 54, 0, -6]/2048);
      | fir1 = dsp.FIRDecimator('DecimationFactor', 2,...
      |                            'CoefficientsDataType', 'Custom',...
      |                            'CustomCoefficientsDataType', numerictype([], 16, 14),...
      |                            'FullPrecisionOverride', false,...
      |                            'OutputDataType', 'Custom',...
      |                            'CustomOutputDataType', numerictype([], 16, 15),...
      |                            'Numerator', [-12, 0, 84, 0, -337, 0, 1008, 0, -2693, 0, 10142, 16384, 10142, 0, -2693, 0, 1008, 0, -337, 0, 84, 0 ,-12]/16384);
      | fir2 = dsp.FIRDecimator('DecimationFactor', 2,...
      |                            'CoefficientsDataType', 'Custom',...
      |                            'CustomCoefficientsDataType', numerictype([], 16, 14),...
      |                            'FullPrecisionOverride', false,...
      |                            'OutputDataType', 'Custom',...
      |                            'CustomOutputDataType', numerictype([], 16, 15),...
      |                            'Numerator', [5, 0, -17, 0, 44, 0, -96, 0, 187, 0, -335, 0, 565, 0, -906, 0, 1401, 0, -2112, 0, 3145, 0, -4723, 0, 7415, 0, -13331, 0, 41526, 65536, 41526, 0, -13331, 0, 7415, 0, -4723, 0, 3145, 0, -2112, 0, 1401, 0, -906, 0, 565, 0, -335, 0, 187, 0, -96, 0, 44, 0, -17, 0, 5]/65536);
      | switch get_param(gcb, 'decim')
      |     case '1x'
      |         if ~strcmp(get_param([gcb, '/FIR 0'], 'Commented'), 'through')
      |             set_param([gcb, '/FIR 0'],'Commented','through');
      |         end
      |         
      |         if ~strcmp(get_param([gcb, '/FIR 1'], 'Commented'), 'through')
      |             set_param([gcb, '/FIR 1'],'Commented','through');
      |         end
      |         
      |         if ~strcmp(get_param([gcb, '/FIR 2'], 'Commented'), 'through')
      |             set_param([gcb, '/FIR 2'],'Commented','through');
      |         end
      |             
      |     case '2x'
      |         if ~strcmp(get_param([gcb, '/FIR 0'], 'Commented'), 'off')
      |             set_param([gcb, '/FIR 0'],'Commented','off');
      |         end
      |         
      |         if ~strcmp(get_param([gcb, '/FIR 1'], 'Commented'), 'through')
      |             set_param([gcb, '/FIR 1'],'Commented','through');
      |         end
      |         
      |         if ~strcmp(get_param([gcb, '/FIR 2'], 'Commented'), 'through')
      |             set_param([gcb, '/FIR 2'],'Commented','through');
      |         end
      | 
      |     case '4x'
      |         if ~strcmp(get_param([gcb, '/FIR 0'], 'Commented'), 'off')
      |             set_param([gcb, '/FIR 0'],'Commented','off');
      |         end
      |         
      |         if ~strcmp(get_param([gcb, '/FIR 1'], 'Commented'), 'off')
      |             set_param([gcb, '/FIR 1'],'Commented','off');
      |         end
      |         
      |         if ~strcmp(get_param([gcb, '/FIR 2'], 'Commented'), 'through')
      |             set_param([gcb, '/FIR 2'],'Commented','through');
      |         end
      |         
      |     case '8x'
      |         if ~strcmp(get_param([gcb, '/FIR 0'], 'Commented'), 'off')
      |             set_param([gcb, '/FIR 0'],'Commented','off');
      |         end
      |         
      |         if ~strcmp(get_param([gcb, '/FIR 1'], 'Commented'), 'off')
      |             set_param([gcb, '/FIR 1'],'Commented','off');
      |         end
      |         
      |         if ~strcmp(get_param([gcb, '/FIR 2'], 'Commented'), 'off')
      |             set_param([gcb, '/FIR 2'],'Commented','off');
      |         end
      | 
      | end
      mask TypeOptions decim: 1x | 2x | 4x | 8x
      mask DialogControl DescGroupVar Prompt: RF-DAC Interpolation Filter
      mask DialogControl DescTextVar Prompt: This block simulates the RF-DAC interpolation stage using the same coefficients stored in the interpolation filters.
      mask DialogControl ParameterGroupVar Prompt: Main
  NCO and Mixer : Subsystem
  RF-ADC : Subsystem
  SSR Converter RF-ADC : Subsystem
  Valid Real : Outport  VectorParamsAs1DForOutWhenUnconnected=off
  Valid Imag : Outport  Port=2  VectorParamsAs1DForOutWhenUnconnected=off
  Data Real : Outport  Port=3  VectorParamsAs1DForOutWhenUnconnected=off
  Data Imag : Outport  Port=4  VectorParamsAs1DForOutWhenUnconnected=off
  wires:
  SSR Converter RF-ADC/2(Valid Imag) -> Valid Imag/1
  SSR Converter RF-ADC/1(Valid Real) -> Valid Real/1
  SSR Converter RF-ADC/3(Real Out) -> Data Real/1
  SSR Converter RF-ADC/4(Imag Out) -> Data Imag/1
  Complex to Real-Imag/2 -> SSR Converter RF-ADC/2(Imag In)
  Complex to Real-Imag/1 -> SSR Converter RF-ADC/1(Real In)
  Decimation Filter/1(Data Out) -> Complex to Real-Imag/1
  Data In/1 -> RF-ADC/1(Data In)
  RF-ADC/1(Data Out) -> NCO and Mixer/1(Data In)
  NCO and Mixer/1(Data Out) -> Decimation Filter/1(Data In)

== system mw_spectrumanalyser/Stimulus and Channel/Channel/RF-DAC ==
  Valid : Inport
  Data : Inport  Port=2
  Interpolation Filter : Subsystem  mask{interp=4x}
      mask prompts: interp "Interpolation Factor:"
      mask init:
      | fir0 = dsp.FIRInterpolator('InterpolationFactor', 2,...
      |                            'CoefficientsDataType', 'Custom',...
      |                            'CustomCoefficientsDataType', numerictype([], 16, 14),...
      |                            'FullPrecisionOverride', false,...
      |                            'OutputDataType', 'Custom',...
      |                            'CustomOutputDataType', numerictype([], 16, 15),...
      |                            'Numerator', [-6, 0 54, 0, -254, 0, 1230, 2048, 1230, 0, -254, 0, 54, 0, -6]/(2048));
      | fir1 = dsp.FIRInterpolator('InterpolationFactor', 2,...
      |                            'CoefficientsDataType', 'Custom',...
      |                            'CustomCoefficientsDataType', numerictype([], 16, 14),...
      |                            'FullPrecisionOverride', false,...
      |                            'OutputDataType', 'Custom',...
      |                            'CustomOutputDataType', numerictype([], 16, 15),...
      |                            'Numerator', [-12, 0, 84, 0, -337, 0, 1008, 0, -2693, 0, 10142, 16384, 10142, 0, -2693, 0, 1008, 0, -337, 0, 84, 0 ,-12]/(16384));
      | fir2 = dsp.FIRInterpolator('InterpolationFactor', 2,...
      |                            'CoefficientsDataType', 'Custom',...
      |                            'CustomCoefficientsDataType', numerictype([], 16, 14),...
      |                            'FullPrecisionOverride', false,...
      |                            'OutputDataType', 'Custom',...
      |                            'CustomOutputDataType', numerictype([], 16, 15),...
      |                            'Numerator', [5, 0, -17, 0, 44, 0, -96, 0, 187, 0, -335, 0, 565, 0, -906, 0, 1401, 0, -2112, 0, 3145, 0, -4723, 0, 7415, 0, -13331, 0, 41526, 65536, 41526, 0, -13331, 0, 7415, 0, -4723, 0, 3145, 0, -2112, 0, 1401, 0, -906, 0, 565, 0, -335, 0, 187, 0, -96, 0, 44, 0, -17, 0, 5]/(65536));
      | switch get_param(gcb, 'interp')
      |     case '1x'
      |         if ~strcmp(get_param([gcb, '/FIR 0'], 'Commented'), 'through')
      |             set_param([gcb, '/FIR 0'],'Commented','through');
      |         end
      |         
      |         if ~strcmp(get_param([gcb, '/FIR 1'], 'Commented'), 'through')
      |             set_param([gcb, '/FIR 1'],'Commented','through');
      |         end
      |         
      |         if ~strcmp(get_param([gcb, '/FIR 2'], 'Commented'), 'through')
      |             set_param([gcb, '/FIR 2'],'Commented','through');
      |         end
      |             
      |     case '2x'
      |         if ~strcmp(get_param([gcb, '/FIR 0'], 'Commented'), 'through')
      |             set_param([gcb, '/FIR 0'],'Commented','through');
      |         end
      |         
      |         if ~strcmp(get_param([gcb, '/FIR 1'], 'Commented'), 'through')
      |             set_param([gcb, '/FIR 1'],'Commented','through');
      |         end
      |         
      |         if ~strcmp(get_param([gcb, '/FIR 2'], 'Commented'), 'off')
      |             set_param([gcb, '/FIR 2'],'Commented','off');
      |         end
      | 
      |     case '4x'
      |         if ~strcmp(get_param([gcb, '/FIR 0'], 'Commented'), 'through')
      |             set_param([gcb, '/FIR 0'],'Commented','through');
      |         end
      |         
      |         if ~strcmp(get_param([gcb, '/FIR 1'], 'Commented'), 'off')
      |             set_param([gcb, '/FIR 1'],'Commented','off');
      |         end
      |         
      |         if ~strcmp(get_param([gcb, '/FIR 2'], 'Commented'), 'off')
      |             set_param([gcb, '/FIR 2'],'Commented','off');
      |         end
      |         
      |     case '8x'
      |         if ~strcmp(get_param([gcb, '/FIR 0'], 'Commented'), 'off')
      |             set_param([gcb, '/FIR 0'],'Commented','off');
      |         end
      |         
      |         if ~strcmp(get_param([gcb, '/FIR 1'], 'Commented'), 'off')
      |             set_param([gcb, '/FIR 1'],'Commented','off');
      |         end
      |         
      |         if ~strcmp(get_param([gcb, '/FIR 2'], 'Commented'), 'off')
      |             set_param([gcb, '/FIR 2'],'Commented','off');
      |         end
      | 
      | end
      mask TypeOptions interp: 1x | 2x | 4x | 8x
      mask DialogControl DescGroupVar Prompt: RF-DAC Interpolation Filter
      mask DialogControl DescTextVar Prompt: This block simulates the RF-DAC interpolation stage using the same coefficients stored in the interpolation filters.
      mask DialogControl ParameterGroupVar Prompt: Main
  NCO and Mixer : Subsystem
  RF-DAC : Subsystem
  SSR Converter RF-DAC : Subsystem
  Data Out : Outport  VectorParamsAs1DForOutWhenUnconnected=off
  wires:
  SSR Converter RF-DAC/1(Data Out) -> Interpolation Filter/1(Data In)
  Valid/1 -> SSR Converter RF-DAC/1(Valid)
  Data/1 -> SSR Converter RF-DAC/2(Data)
  Interpolation Filter/1(Data Out) -> NCO and Mixer/1(Data In)
  NCO and Mixer/1(Data Out) -> RF-DAC/1(Data In)
  RF-DAC/1(Data Out) -> Data Out/1
